simulink model "QuadrotorSimulink_w_memory_error"  (R2020a)
settings: Solver=FixedStepAuto  StartTime=0.0  StopTime=options.T_train  FixedStep=options.dt  RelTol=1e-6
undefined symbols (not defined in the file or in its folder): options, Quad
libraries: neural x67, simulink x2
(part 5 of 5)

== system QuadrotorSimulink_w_memory_error/NN/Layer 3/Delays 1 ==
  "p{3}" : Inport  PortDimensions=30
      mask Display: e = 0.06;c1 = [120 230 180]/255;c2 = ([120 230 180]+0)/(256+128);c3 = ([120 230 180]+128)/(256+128);patch([0 1 1 0],[0 0 1 1],c1);patch([0 1 1 1-e 1-e 0+e],[0 0 1 1-e 0+e 0+e],c2);patch([0 0 1 1-e 0+e 0+e],[0 1 1 1-e 1-e 0+e],c3);plot([0 1 1 0 0],[0 0 1 1 0]);
  mux : Mux  Inputs=1
      mask Display: e = 0.06;c1 = [120 150 230]/255;c2 = ([120 150 230]+0)/383;c3 = ([120 150 230]+128)/383;patch([0 1 1 0],[0 0 1 1],c1);patch([0 1 1 1-e 1-e 0+e],[0 0 1 1-e 0+e 0+e],c2);patch([0 0 1 1-e 0+e 0+e],[0 1 1 1-e 1-e 0+e],c3);plot([0 1 1 0 0],[0 0 1 1 0]);disp('Mux')
  "pd{3,2}" : Outport
      mask Display: e = 0.06;c1 = [120 230 180]/255;c2 = ([120 230 180]+0)/(256+128);c3 = ([120 230 180]+128)/(256+128);patch([0 1 1 0],[0 0 1 1],c1);patch([0 1 1 1-e 1-e 0+e],[0 0 1 1-e 0+e 0+e],c2);patch([0 0 1 1-e 0+e 0+e],[0 1 1 1-e 1-e 0+e],c3);plot([0 1 1 0 0],[0 0 1 1 0]);
  wires:
  "p{3}"/1 -> mux/1
  mux/1 -> "pd{3,2}"/1

== system QuadrotorSimulink_w_memory_error/NN/Layer 3/LW{3,2} ==
  "ad{3,2}" : Inport  PortDimensions=30
      mask Display: e = 0.06;c1 = [120 230 180]/255;c2 = ([120 230 180]+0)/(256+128);c3 = ([120 230 180]+128)/(256+128);patch([0 1 1 0],[0 0 1 1],c1);patch([0 1 1 1-e 1-e 0+e],[0 0 1 1-e 0+e 0+e],c2);patch([0 0 1 1-e 0+e 0+e],[0 1 1 1-e 1-e 0+e],c3);plot([0 1 1 0 0],[0 0 1 1 0]);
  "IW{3,2}(1,:)'" : Constant  Value=[-0.01407572277703103384716154522493525291793048381805419921875;-0.10789950346018802040948258991193142719566822052001953125;-0.9607172439475373248995992980781011283397674560546875;-1.0925042103762854228676815182552672922611236572265625;1.2337080303882839160678486223332583904266357421875;0.38341285920569012635183980819419957697391510009765625;-0.303510064774958288058570587963913567364215850830078125;0.70329362149470486809121894111740402877330780029296875;0.5083236822901497919957591875572688877582550048828125;0.146213222999473313468143942372989840805530548095703125;-0.29085476660379983027127082095830701291561126708984375;-1.2370619196013683538382110782549716532230377197265625;1.347101985952784186650887932046316564083099365234375;-0.251136327801185943453532445346354506909847259521484375;-0.277051781857630186056695720253628678619861602783203125;-0.77866837608694605687986722841742448508739471435546875;0.39081883710680731525144437910057604312896728515625;0.1533755135644482014978251527281827293336391448974609375;-0.2030836979208179016165303210073034279048442840576171875;-0.1996379140942204644115776090984581969678401947021484375;-0.5014682298319559361488018112140707671642303466796875;-1.980912905092413023311337383347563445568084716796875;-1.005155993575960859942597380722872912883758544921875;0.31360370757203737124285680692992173135280609130859375;0.196320126054053079034389384105452336370944976806640625;0.30238487772676603260180172583204694092273712158203125;-0.8295582084721591087372871697880327701568603515625;0.044549700970445811620823661769463797099888324737548828125;-1.6118033555058719485941765015013515949249267578125;-1.354777770085710653091837230022065341472625732421875]
      mask Display: e = 0.06;c1 = [120 150 230]/255;c2 = ([120 150 230]+0)/383;c3 = ([120 150 230]+128)/383;patch([0 1 1 0],[0 0 1 1],c1);patch([0 1 1 1-e 1-e 0+e],[0 0 1 1-e 0+e 0+e],c2);patch([0 0 1 1-e 0+e 0+e],[0 1 1 1-e 1-e 0+e],c3);plot([0 1 1 0 0],[0 0 1 1 0]);disp('weights');
  "IW{3,2}(2,:)'" : Constant  Value=[-0.461658293296777377801021202685660682618618011474609375;-0.0491842302840182765688581412177882157266139984130859375;0.176146994005770995972426362641272135078907012939453125;0.7086988770334434750708396677509881556034088134765625;0.57998224796869379815689171664416790008544921875;-0.312180220078959014262665050409850664436817169189453125;-0.43859664523234498378911894178600050508975982666015625;-1.234729997046596139398388913832604885101318359375;0.178682837191655730091355280819698236882686614990234375;0.612135896133761736592759916675277054309844970703125;-0.64289812292079495659180565780843608081340789794921875;0.1657930327130838488169928268689545802772045135498046875;-0.278652326598373745181191907249740324914455413818359375;-0.172415522114090558059018576386733911931514739990234375;-0.5864590594781162735671387054026126861572265625;0.57425976765660424749881940442719496786594390869140625;-0.938826314420332597165952392970211803913116455078125;0.75582310300437860473010687201167456805706024169921875;-0.189814972102107459850373061271966435015201568603515625;-0.37260322949215718413285003407509066164493560791015625;0.53221681442357127167497310438193380832672119140625;0.1552461304229036109791906028476660139858722686767578125;0.25435917191181445229375412964145652949810028076171875;-0.09469322986400728614508892633239156566560268402099609375;0.32867410504314487074140060940408147871494293212890625;0.62063580054503830751855275593698024749755859375;0.397797204442776830557448874969850294291973114013671875;0.16299943409629713553243846035911701619625091552734375;-0.39321017351359321967407822739914990961551666259765625;-0.2849471273026040751830123554100282490253448486328125]
      mask Display: e = 0.06;c1 = [120 150 230]/255;c2 = ([120 150 230]+0)/383;c3 = ([120 150 230]+128)/383;patch([0 1 1 0],[0 0 1 1],c1);patch([0 1 1 1-e 1-e 0+e],[0 0 1 1-e 0+e 0+e],c2);patch([0 0 1 1-e 0+e 0+e],[0 1 1 1-e 1-e 0+e],c3);plot([0 1 1 0 0],[0 0 1 1 0]);disp('weights');
  Mux : Mux  Inputs=2
      mask Display: e = 0.06;c1 = [120 150 230]/255;c2 = ([120 150 230]+0)/383;c3 = ([120 150 230]+128)/383;patch([0 1 1 0],[0 0 1 1],c1);patch([0 1 1 1-e 1-e 0+e],[0 0 1 1-e 0+e 0+e],c2);patch([0 0 1 1-e 0+e 0+e],[0 1 1 1-e 1-e 0+e],c3);plot([0 1 1 0 0],[0 0 1 1 0]);disp('Mux');
  dotprod1 : neural/Weight Functions/dotprod
  dotprod2 : neural/Weight Functions/dotprod
  "lz{3,2}" : Outport
      mask Display: e = 0.06;c1 = [120 230 180]/255;c2 = ([120 230 180]+0)/(256+128);c3 = ([120 230 180]+128)/(256+128);patch([0 1 1 0],[0 0 1 1],c1);patch([0 1 1 1-e 1-e 0+e],[0 0 1 1-e 0+e 0+e],c2);patch([0 0 1 1-e 0+e 0+e],[0 1 1 1-e 1-e 0+e],c3);plot([0 1 1 0 0],[0 0 1 1 0]);
  wires:
  "IW{3,2}(1,:)'"/1 -> dotprod1/1
  "ad{3,2}"/1 -> dotprod1/2, dotprod2/2
  dotprod1/1 -> Mux/1
  "IW{3,2}(2,:)'"/1 -> dotprod2/1
  dotprod2/1 -> Mux/2
  Mux/1 -> "lz{3,2}"/1
